simulink model "bangbang"  (R2019b)
settings: Solver=VariableStepAuto  StartTime=0.0  StopTime=horizon  RelTol=1e-3
undefined symbols (not defined in the file or in its folder): J, usat, x0, xdot0
libraries: simulink x1
settings Model: Creator=d.alazard  LastModifiedBy=d.alazard

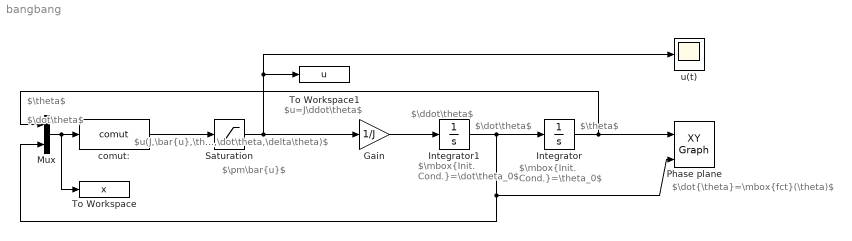
== system bangbang ==
  note: $\mbox{Init. Cond.}=\dot\theta_0$
  note: $\pm\bar{u}$
  note: $u(J,\bar{u},\theta,\dot\theta,\delta\theta)$
  note: $\dot{\theta}=\mbox{fct}(\theta)$
  note: $\theta$
  note: $\dot\theta$
  note: $\ddot\theta$
  note: $u=J\ddot\theta$
  note: $\theta$
  note: $\dot\theta$
  note: $\mbox{Init. Cond.}=\theta_0$
  Gain : Gain  Gain=1/J
  Integrator : Integrator  InitialCondition=x0
  Integrator1 : Integrator  InitialCondition=xdot0
  Mux : Mux  Inputs=2
  Phase plane : simulink/Sinks/XY Graph  xmin=min(-1,-2*abs(x0))  xmax=max(1,2*abs(x0))  ymin=min(-1,-3*abs(xdot0))  ymax=max(1,3*abs(xdot0))  st=-1
  Saturation : Saturate  UpperLimit=usat  LowerLimit=-usat
  To Workspace : ToWorkspace  VariableName=x  SaveFormat=Structure With Time  SampleTime=-1
  To Workspace1 : ToWorkspace  VariableName=u  SaveFormat=Structure With Time  SampleTime=-1
  comut: : MATLABFcn  MATLABFcn=comut  OutputDimensions=1
  u(t) : Scope
  wires:
  Gain/1 -> Integrator1/1
  Integrator1/1 -> Mux/2, Phase plane/2, Integrator/1
  Saturation/1 -> Gain/1, To Workspace1/1, u(t)/1
  comut:/1 -> Saturation/1
  Mux/1 -> To Workspace/1, comut:/1
  Integrator/1 -> Phase plane/1, Mux/1
